simulink model "DynamicCompensator"  (R2023a)
settings: Solver=VariableStepAuto  StartTime=0.0  StopTime=200  RelTol=1e-3
values from neighbouring files (symbols this model uses):
  AL = A-L*C    [Script_Dirigibile.m]
  BL = [B L]    [Script_Dirigibile.m]
  C = C(1,:)    [Script_Dirigibile.m]
  K = acker(A, B, [-0.25 -0.42 -0.037])    [Script_Dirigibile.m]
  x0_tilde = [x0(1)-xeq(1) x0(2)-xeq(2) x0(3)-xeq(3)]    [Script_Dirigibile.m]
  yeq = x_eq    [Script_Dirigibile.m]
undefined symbols (not defined in the file or in its folder): A, B
settings Model: Creator=giuco  LastModifiedBy=giuco

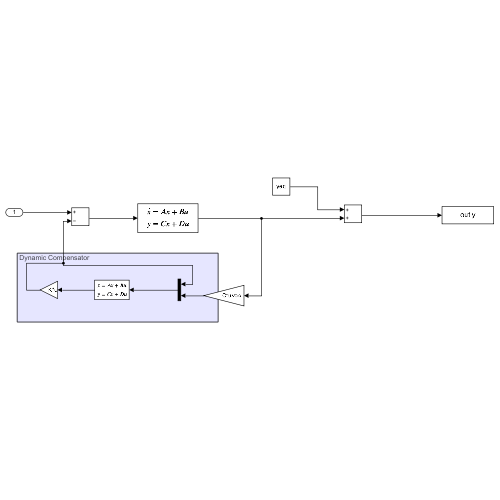
[thumbnail: Simulink's stored preview of the top-level diagram]
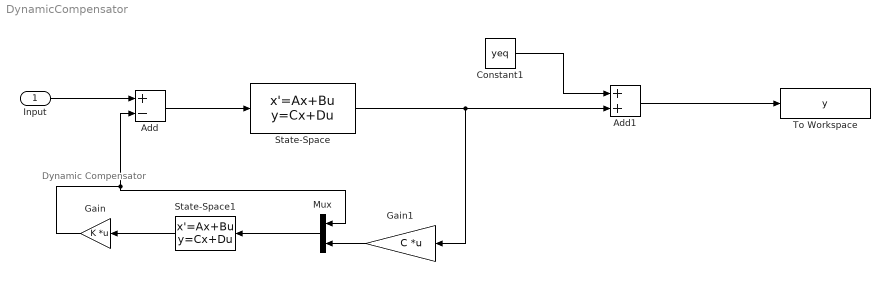
== system DynamicCompensator ==
  note: Dynamic Compensator
  Input : Inport
  Add : Sum  Inputs=+-
  Add1 : Sum
  Constant1 : Constant  Value=yeq
  Gain : Gain  Gain=K  Multiplication=Matrix(K*u)
  Gain1 : Gain  Gain=C  Multiplication=Matrix(K*u) (u vector)
  Mux : Mux  Inputs=2
  State-Space : StateSpace  A=A  B=B  C=eye(3)  D=zeros(3,1)  InitialCondition=x0_tilde
  State-Space1 : StateSpace  A=AL  B=BL  C=eye(3)  D=zeros(3,2)  InitialCondition=[0;0;0]
  To Workspace : ToWorkspace  VariableName=y  SaveFormat=Timeseries  SampleTime=-1
  wires:
  Add/1 -> State-Space/1
  State-Space/1 -> Add1/2, Gain1/1
  State-Space1/1 -> Gain/1
  Gain/1 -> Mux/1, Add/2
  Mux/1 -> State-Space1/1
  Gain1/1 -> Mux/2
  Add1/1 -> To Workspace/1
  Constant1/1 -> Add1/1
  Input/1 -> Add/1
